simulink model "simon_internal_pipelined_interleaved"  (R2015b)
settings: Solver=FixedStepDiscrete  SolverMode=SingleTasking  StartTime=0.0  StopTime=5^-4  RelTol=1e-3
undefined symbols (not defined in the file or in its folder): a, b
libraries: shlslibv1 x86
settings Model: synDspstartup=OK  Creator=ASUAD\pgali  LastModifiedBy=vchand32
settings DataIOCC: SaveOutput=off  SignalLogging=off  SaveTime=off
settings OptimizationCC: DefaultParameterBehavior=Inlined
settings DebuggingCC: AlgebraicLoopMsg=error  InheritedTsInSrcMsg=none

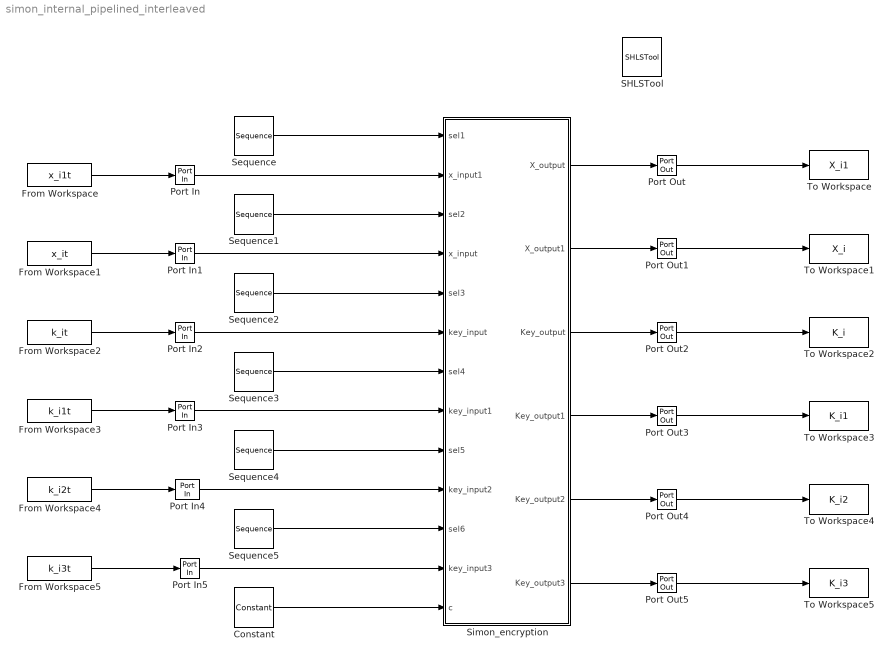
== system simon_internal_pipelined_interleaved ==
  Constant : shlslibv1/Sources/Constant  syn_cst_val=65532  syn_cst_format=Automatic  syn_cst_wl=1  syn_cst_fl=0  syn_cst_dt=unsigned  syn_cst_rnd=on  syn_cst_st=1/645e6  synBlockType=primitive  synLatency=0  synBlockId=15
  From Workspace : FromWorkspace  VariableName=x_i1t  SampleTime=0
  From Workspace1 : FromWorkspace  VariableName=x_it  SampleTime=0
  From Workspace2 : FromWorkspace  VariableName=k_it  SampleTime=0
  From Workspace3 : FromWorkspace  VariableName=k_i1t  SampleTime=0
  From Workspace4 : FromWorkspace  VariableName=k_i2t  SampleTime=0
  From Workspace5 : FromWorkspace  VariableName=k_i3t  SampleTime=0
  Port In{,1..5} (6 alike) : shlslibv1/Ports & Subsystems/Port In  syn_out_wl=16  syn_out_fl=0  syn_out_dt=unsigned  syn_out_st=1/645e6  syn_capture=on  syn_register=on  syn_out_sat=off  syn_out_rnd=on  synBlockType=port  synLatency=1  synBlockId=0
  Port Out{,1..5} (6 alike) : shlslibv1/Ports & Subsystems/Port Out  syn_capture=on  syn_register=on  synBlockType=port  synLatency=1  synBlockId=1
  SHLSTool : shlslibv1/SHLSTool  synBlockType=tool  syn_dsp_mode=FPGA
  Sequence{,1..5} (6 alike) : shlslibv1/Sources/Sequence  syn_seq_vec=[0 0 0 0 1 1 1 1 1 1 1 1 1 1 1 1 1 1 1 1 1 1 1 1 1 1 1 1 1 1 1 1 1 1 1 1 1 1 1 1 1 1 1 1 1 1 1 1 1 1 1 1 1 1 1 1 1 1 1 1 1 1 1 1 1 1 1 1 1 1 1 1 1 1 1 1 1 1 1 1 1 1 1 1 1 1 1 1 1 1 1 1 1 1 1 1 1 1 1 1 1 1 1 1 1 1 1 1 1 1 1 1 1 1 1 1 1 1 1 1 1 1 1 1 1 1 1 1]  syn_seq_wl=1  syn_seq_fl=0  syn_seq_dt=unsigned  syn_rst_port=off  syn_en_port=off  syn_seq_st=1/645e6  synBlockType=custom  synLatency=1
  "Simon_encryption " : Subsystem
  To Workspace : ToWorkspace  VariableName=X_i1  SaveFormat=Structure With Time  SampleTime=-1
  To Workspace1 : ToWorkspace  VariableName=X_i  SaveFormat=Structure With Time  SampleTime=-1
  To Workspace2 : ToWorkspace  VariableName=K_i  SaveFormat=Structure With Time  SampleTime=-1
  To Workspace3 : ToWorkspace  VariableName=K_i1  SaveFormat=Structure With Time  SampleTime=-1
  To Workspace4 : ToWorkspace  VariableName=K_i2  SaveFormat=Structure With Time  SampleTime=-1
  To Workspace5 : ToWorkspace  VariableName=K_i3  SaveFormat=Structure With Time  SampleTime=-1
  wires:
  From Workspace1/1 -> Port In1/1
  From Workspace2/1 -> Port In2/1
  "Simon_encryption "/1(X_output) -> Port Out/1
  "Simon_encryption "/2(X_output1) -> Port Out1/1
  "Simon_encryption "/3(Key_output) -> Port Out2/1
  "Simon_encryption "/4(Key_output1) -> Port Out3/1
  "Simon_encryption "/5(Key_output2) -> Port Out4/1
  "Simon_encryption "/6(Key_output3) -> Port Out5/1
  From Workspace/1 -> Port In/1
  Constant/1 -> "Simon_encryption "/13(c)
  From Workspace3/1 -> Port In3/1
  From Workspace4/1 -> Port In4/1
  From Workspace5/1 -> Port In5/1
  Port In/1 -> "Simon_encryption "/2(x_input1)
  Port In1/1 -> "Simon_encryption "/4(x_input)
  Port In2/1 -> "Simon_encryption "/6(key_input)
  Port In3/1 -> "Simon_encryption "/8(key_input1)
  Port In4/1 -> "Simon_encryption "/10(key_input2)
  Port In5/1 -> "Simon_encryption "/12(key_input3)
  Port Out/1 -> To Workspace/1
  Port Out1/1 -> To Workspace1/1
  Port Out3/1 -> To Workspace3/1
  Port Out4/1 -> To Workspace4/1
  Port Out5/1 -> To Workspace5/1
  Port Out2/1 -> To Workspace2/1
  Sequence/1 -> "Simon_encryption "/1(sel1)
  Sequence1/1 -> "Simon_encryption "/3(sel2)
  Sequence2/1 -> "Simon_encryption "/5(sel3)
  Sequence3/1 -> "Simon_encryption "/7(sel4)
  Sequence4/1 -> "Simon_encryption "/9(sel5)
  Sequence5/1 -> "Simon_encryption "/11(sel6)

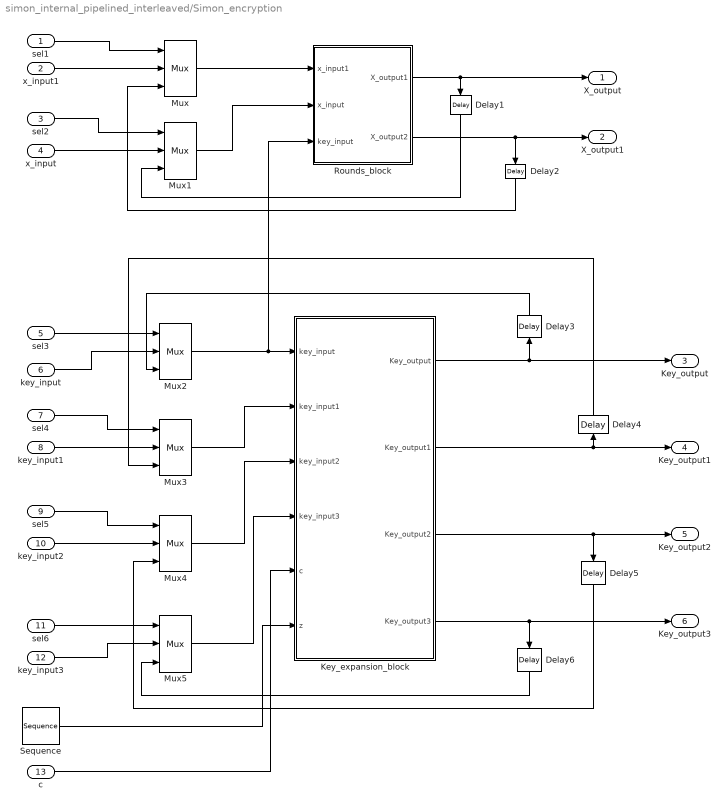
== system simon_internal_pipelined_interleaved/Simon_encryption  ==
  sel1 : Inport
  x_input1 : Inport  Port=2
  sel2 : Inport  Port=3
  x_input : Inport  Port=4
  sel3 : Inport  Port=5
  key_input : Inport  Port=6
  sel4 : Inport  Port=7
  key_input1 : Inport  Port=8
  sel5 : Inport  Port=9
  key_input2 : Inport  Port=10
  sel6 : Inport  Port=11
  key_input3 : Inport  Port=12
  c : Inport  Port=13
  Delay{1..6} (6 alike) : shlslibv1/Memories/Delay  syn_delay_val=1  synBlockType=primitive  synLatency=1  synBlockId=104
  Key_expansion_block : Subsystem
  Mux{,1..5} (6 alike) : shlslibv1/Signal Operations/Mux  syn_in_nb=2  syn_out_f=Full Precision  syn_out_wl=16  syn_out_fl=8  syn_out_dt=signed  syn_en_se=off  synBlockType=primitive  synLatency=0  synBlockId=16
  Rounds_block : Subsystem
  Sequence : shlslibv1/Sources/Sequence  syn_seq_vec=[1 1 1 1 1 1 1 1 1 1 1 1 1 1 1 1 1 1 1 1 0 0 0 0 1 1 1 1 0 0 0 0 0 0 0 0 0 0 0 0 1 1 1 1 0 0 0 0 0 0 0 0 1 1 1 1 0 0 0 0 1 1 1 1 0 0 0 0 1 1 1 1 1 1 1 1 0 0 0 0 0 0 0 0 0 0 0 0 0 0 0 0 1 1 1 1 1 1 1 1 1 1 1 1 0 0 0 0 0 0 0 0 1 1 1 1 1 1 1 1 0 0 0 0 0 0 0 0]  syn_seq_wl=16  syn_seq_fl=0  syn_seq_dt=unsigned  syn_rst_port=off  syn_en_port=off  syn_seq_st=-1  synBlockType=custom  synLatency=1
  X_output : Outport
  X_output1 : Outport  Port=2
  Key_output : Outport  Port=3
  Key_output1 : Outport  Port=4
  Key_output2 : Outport  Port=5
  Key_output3 : Outport  Port=6
  wires:
  sel1/1 -> Mux/1
  x_input1/1 -> Mux/2
  Rounds_block/1(X_output1) -> X_output/1, Delay1/1
  Rounds_block/2(X_output2) -> Delay2/1, X_output1/1
  sel2/1 -> Mux1/1
  x_input/1 -> Mux1/2
  sel3/1 -> Mux2/1
  sel4/1 -> Mux3/1
  key_input1/1 -> Mux3/2
  sel5/1 -> Mux4/1
  key_input2/1 -> Mux4/2
  sel6/1 -> Mux5/1
  key_input3/1 -> Mux5/2
  Key_expansion_block/2(Key_output1) -> Delay4/1, Key_output1/1
  Key_expansion_block/3(Key_output2) -> Delay5/1, Key_output2/1
  Key_expansion_block/4(Key_output3) -> Delay6/1, Key_output3/1
  c/1 -> Key_expansion_block/5(c)
  key_input/1 -> Mux2/2
  Key_expansion_block/1(Key_output) -> Delay3/1, Key_output/1
  Mux/1 -> Rounds_block/1(" x_input1")
  Mux1/1 -> Rounds_block/2(x_input)
  Mux2/1 -> Rounds_block/3(key_input), Key_expansion_block/1(key_input)
  Mux3/1 -> Key_expansion_block/2(key_input1)
  Mux4/1 -> Key_expansion_block/3(key_input2)
  Mux5/1 -> Key_expansion_block/4(key_input3)
  Delay1/1 -> Mux1/3
  Delay6/1 -> Mux5/3
  Delay5/1 -> Mux4/3
  Delay4/1 -> Mux3/3
  Delay3/1 -> Mux2/3
  Sequence/1 -> Key_expansion_block/6(z)
  Delay2/1 -> Mux/3

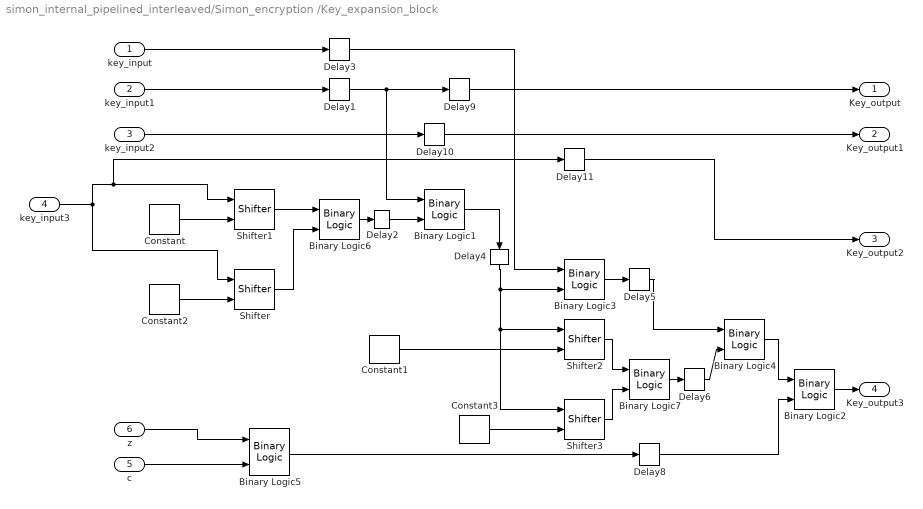
== system simon_internal_pipelined_interleaved/Simon_encryption /Key_expansion_block ==
  key_input : Inport
  key_input1 : Inport  Port=2
  key_input2 : Inport  Port=3
  key_input3 : Inport  Port=4
  c : Inport  Port=5
  z : Inport  Port=6
  Binary Logic{1..5} (5 alike) : shlslibv1/Math Functions/Binary Logic  syn_binlog_exp=a^b  synBlockType=primitive  synLatency=0  synBlockId=13
  Binary Logic6 : shlslibv1/Math Functions/Binary Logic  syn_binlog_exp=a|b  synBlockType=primitive  synLatency=0  synBlockId=13
  Binary Logic7 : shlslibv1/Math Functions/Binary Logic  syn_binlog_exp=a|b  synBlockType=primitive  synLatency=0  synBlockId=13
  Constant : shlslibv1/Sources/Constant  syn_cst_val=3  syn_cst_format=Specify  syn_cst_wl=4  syn_cst_fl=0  syn_cst_dt=unsigned  syn_cst_rnd=on  syn_cst_st=-1  synBlockType=primitive  synLatency=0  synBlockId=15
  Constant1 : shlslibv1/Sources/Constant  syn_cst_val=1  syn_cst_format=Specify  syn_cst_wl=4  syn_cst_fl=0  syn_cst_dt=unsigned  syn_cst_rnd=on  syn_cst_st=-1  synBlockType=primitive  synLatency=0  synBlockId=15
  Constant2 : shlslibv1/Sources/Constant  syn_cst_val=13  syn_cst_format=Specify  syn_cst_wl=4  syn_cst_fl=0  syn_cst_dt=unsigned  syn_cst_rnd=on  syn_cst_st=-1  synBlockType=primitive  synLatency=0  synBlockId=15
  Constant3 : shlslibv1/Sources/Constant  syn_cst_val=15  syn_cst_format=Specify  syn_cst_wl=4  syn_cst_fl=0  syn_cst_dt=unsigned  syn_cst_rnd=on  syn_cst_st=-1  synBlockType=primitive  synLatency=0  synBlockId=15
  Delay{1..2,4..6} (5 alike) : shlslibv1/Memories/Delay  syn_delay_val=1  synBlockType=primitive  synLatency=1  synBlockId=104
  Delay10 : shlslibv1/Memories/Delay  syn_delay_val=3  synBlockType=primitive  synLatency=3  synBlockId=104
  Delay11 : shlslibv1/Memories/Delay  syn_delay_val=3  synBlockType=primitive  synLatency=3  synBlockId=104
  Delay3 : shlslibv1/Memories/Delay  syn_delay_val=2  synBlockType=primitive  synLatency=2  synBlockId=104
  Delay8 : shlslibv1/Memories/Delay  syn_delay_val=3  synBlockType=primitive  synLatency=3  synBlockId=104
  Delay9 : shlslibv1/Memories/Delay  syn_delay_val=2  synBlockType=primitive  synLatency=2  synBlockId=104
  Shifter : shlslibv1/Math Functions/Shifter  syn_shifter_opr=<<  syn_out_f=Automatic  syn_out_wl=16  syn_out_fl=8  syn_out_dt=signed  synBlockType=primitive  synLatency=0  synBlockId=12
  Shifter1 : shlslibv1/Math Functions/Shifter  syn_shifter_opr=>>  syn_out_f=Automatic  syn_out_wl=16  syn_out_fl=8  syn_out_dt=signed  synBlockType=primitive  synLatency=0  synBlockId=12
  Shifter2 : shlslibv1/Math Functions/Shifter  syn_shifter_opr=>>  syn_out_f=Automatic  syn_out_wl=16  syn_out_fl=8  syn_out_dt=signed  synBlockType=primitive  synLatency=0  synBlockId=12
  Shifter3 : shlslibv1/Math Functions/Shifter  syn_shifter_opr=<<  syn_out_f=Automatic  syn_out_wl=16  syn_out_fl=8  syn_out_dt=signed  synBlockType=primitive  synLatency=0  synBlockId=12
  Key_output : Outport
  Key_output1 : Outport  Port=2
  Key_output2 : Outport  Port=3
  Key_output3 : Outport  Port=4
  wires:
  Binary Logic1/1 -> Delay4/1
  Constant/1 -> Shifter1/2
  Constant1/1 -> Shifter2/2
  Binary Logic2/1 -> Key_output3/1
  key_input/1 -> Delay3/1
  key_input1/1 -> Delay1/1
  z/1 -> Binary Logic5/1
  c/1 -> Binary Logic5/2
  key_input2/1 -> Delay10/1
  key_input3/1 -> Shifter1/1, Delay11/1, Shifter/1
  Binary Logic3/1 -> Delay5/1
  Binary Logic5/1 -> Delay8/1
  Constant2/1 -> Shifter/2
  Shifter1/1 -> Binary Logic6/1
  Shifter/1 -> Binary Logic6/2
  Constant3/1 -> Shifter3/2
  Shifter2/1 -> Binary Logic7/1
  Shifter3/1 -> Binary Logic7/2
  Delay1/1 -> Binary Logic1/1, Delay9/1
  Binary Logic6/1 -> Delay2/1
  Delay2/1 -> Binary Logic1/2
  Delay3/1 -> Binary Logic3/1
  Delay4/1 -> Binary Logic3/2, Shifter2/1, Shifter3/1
  Delay5/1 -> Binary Logic4/1
  Binary Logic7/1 -> Delay6/1
  Delay6/1 -> Binary Logic4/2
  Binary Logic4/1 -> Binary Logic2/1
  Delay8/1 -> Binary Logic2/2
  Delay9/1 -> Key_output/1
  Delay10/1 -> Key_output1/1
  Delay11/1 -> Key_output2/1

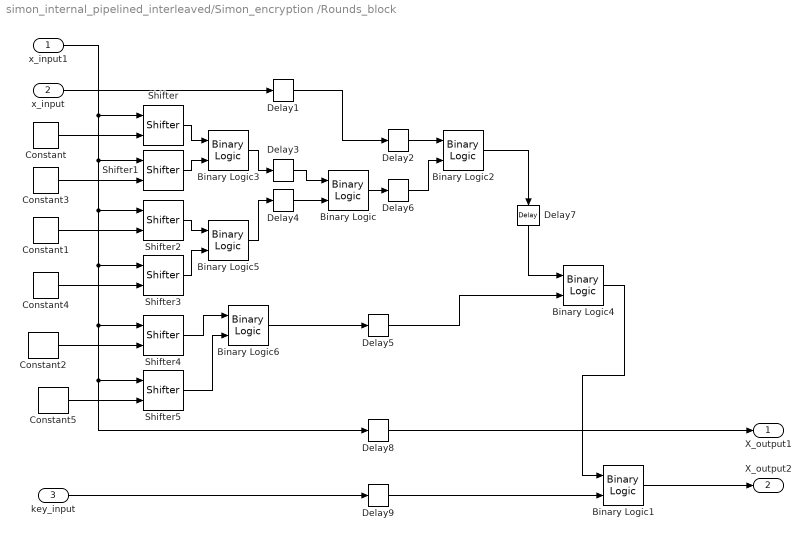
== system simon_internal_pipelined_interleaved/Simon_encryption /Rounds_block ==
  " x_input1" : Inport  OutMin=[0]  OutMax=[0]
  x_input : Inport  Port=2  OutMin=[0]  OutMax=[0]
  key_input : Inport  Port=3  OutMin=[0]  OutMax=[0]
  Binary Logic : shlslibv1/Math Functions/Binary Logic  syn_binlog_exp=a&b  synBlockType=primitive  synLatency=0  synBlockId=13
  Binary Logic1 : shlslibv1/Math Functions/Binary Logic  syn_binlog_exp=a^b  synBlockType=primitive  synLatency=0  synBlockId=13
  Binary Logic2 : shlslibv1/Math Functions/Binary Logic  syn_binlog_exp=a^b  synBlockType=primitive  synLatency=0  synBlockId=13
  Binary Logic3 : shlslibv1/Math Functions/Binary Logic  syn_binlog_exp=a|b  synBlockType=primitive  synLatency=0  synBlockId=13
  Binary Logic4 : shlslibv1/Math Functions/Binary Logic  syn_binlog_exp=a^b  synBlockType=primitive  synLatency=0  synBlockId=13
  Binary Logic5 : shlslibv1/Math Functions/Binary Logic  syn_binlog_exp=a|b  synBlockType=primitive  synLatency=0  synBlockId=13
  Binary Logic6 : shlslibv1/Math Functions/Binary Logic  syn_binlog_exp=a|b  synBlockType=primitive  synLatency=0  synBlockId=13
  Constant : shlslibv1/Sources/Constant  syn_cst_val=1  syn_cst_format=Specify  syn_cst_wl=4  syn_cst_fl=0  syn_cst_dt=unsigned  syn_cst_rnd=on  syn_cst_st=-1  synBlockType=primitive  synLatency=0  synBlockId=15
  Constant1 : shlslibv1/Sources/Constant  syn_cst_val=8  syn_cst_format=Specify  syn_cst_wl=4  syn_cst_fl=0  syn_cst_dt=unsigned  syn_cst_rnd=on  syn_cst_st=-1  synBlockType=primitive  synLatency=0  synBlockId=15
  Constant2 : shlslibv1/Sources/Constant  syn_cst_val=2  syn_cst_format=Specify  syn_cst_wl=4  syn_cst_fl=0  syn_cst_dt=unsigned  syn_cst_rnd=on  syn_cst_st=-1  synBlockType=primitive  synLatency=0  synBlockId=15
  Constant3 : shlslibv1/Sources/Constant  syn_cst_val=15  syn_cst_format=Specify  syn_cst_wl=4  syn_cst_fl=0  syn_cst_dt=unsigned  syn_cst_rnd=on  syn_cst_st=-1  synBlockType=primitive  synLatency=0  synBlockId=15
  Constant4 : shlslibv1/Sources/Constant  syn_cst_val=8  syn_cst_format=Specify  syn_cst_wl=4  syn_cst_fl=0  syn_cst_dt=unsigned  syn_cst_rnd=on  syn_cst_st=-1  synBlockType=primitive  synLatency=0  synBlockId=15
  Constant5 : shlslibv1/Sources/Constant  syn_cst_val=14  syn_cst_format=Specify  syn_cst_wl=4  syn_cst_fl=0  syn_cst_dt=unsigned  syn_cst_rnd=on  syn_cst_st=-1  synBlockType=primitive  synLatency=0  synBlockId=15
  Delay{1..4,6..7} (6 alike) : shlslibv1/Memories/Delay  syn_delay_val=1  synBlockType=primitive  synLatency=1  synBlockId=104
  Delay5 : shlslibv1/Memories/Delay  syn_delay_val=3  synBlockType=primitive  synLatency=3  synBlockId=104
  Delay8 : shlslibv1/Memories/Delay  syn_delay_val=3  synBlockType=primitive  synLatency=3  synBlockId=104
  Delay9 : shlslibv1/Memories/Delay  syn_delay_val=3  synBlockType=primitive  synLatency=3  synBlockId=104
  Shifter : shlslibv1/Math Functions/Shifter  syn_shifter_opr=<<  syn_out_f=Automatic  syn_out_wl=16  syn_out_fl=8  syn_out_dt=signed  synBlockType=primitive  synLatency=0  synBlockId=12
  Shifter1 : shlslibv1/Math Functions/Shifter  syn_shifter_opr=>>  syn_out_f=Automatic  syn_out_wl=16  syn_out_fl=8  syn_out_dt=signed  synBlockType=primitive  synLatency=0  synBlockId=12
  Shifter2 : shlslibv1/Math Functions/Shifter  syn_shifter_opr=<<  syn_out_f=Automatic  syn_out_wl=16  syn_out_fl=8  syn_out_dt=signed  synBlockType=primitive  synLatency=0  synBlockId=12
  Shifter3 : shlslibv1/Math Functions/Shifter  syn_shifter_opr=>>  syn_out_f=Automatic  syn_out_wl=16  syn_out_fl=8  syn_out_dt=signed  synBlockType=primitive  synLatency=0  synBlockId=12
  Shifter4 : shlslibv1/Math Functions/Shifter  syn_shifter_opr=<<  syn_out_f=Automatic  syn_out_wl=16  syn_out_fl=8  syn_out_dt=signed  synBlockType=primitive  synLatency=0  synBlockId=12
  Shifter5 : shlslibv1/Math Functions/Shifter  syn_shifter_opr=>>  syn_out_f=Automatic  syn_out_wl=16  syn_out_fl=8  syn_out_dt=signed  synBlockType=primitive  synLatency=0  synBlockId=12
  X_output1 : Outport
  X_output2 : Outport  Port=2
  wires:
  Binary Logic2/1 -> Delay7/1
  Constant/1 -> Shifter/2
  Constant1/1 -> Shifter2/2
  Binary Logic1/1 -> X_output2/1
  x_input/1 -> Delay1/1
  " x_input1"/1 -> Shifter/1, Shifter1/1, Shifter2/1, Shifter3/1, Shifter4/1, Delay8/1, Shifter5/1
  key_input/1 -> Delay9/1
  Constant3/1 -> Shifter1/2
  Shifter/1 -> Binary Logic3/1
  Shifter1/1 -> Binary Logic3/2
  Constant4/1 -> Shifter3/2
  Shifter2/1 -> Binary Logic5/1
  Shifter3/1 -> Binary Logic5/2
  Constant2/1 -> Shifter4/2
  Shifter4/1 -> Binary Logic6/1
  Constant5/1 -> Shifter5/2
  Shifter5/1 -> Binary Logic6/2
  Binary Logic6/1 -> Delay5/1
  Delay1/1 -> Delay2/1
  Binary Logic3/1 -> Delay3/1
  Binary Logic5/1 -> Delay4/1
  Delay4/1 -> Binary Logic/2
  Delay2/1 -> Binary Logic2/1
  Binary Logic/1 -> Delay6/1
  Delay6/1 -> Binary Logic2/2
  Delay5/1 -> Binary Logic4/2
  Delay7/1 -> Binary Logic4/1
  Delay9/1 -> Binary Logic1/2
  Delay3/1 -> Binary Logic/1
  Delay8/1 -> X_output1/1
  Binary Logic4/1 -> Binary Logic1/1
